simulink model "AMI_2_2_2"  (R2024b)
settings: Solver=FixedStepAuto  StartTime=0.0  StopTime=inf  FixedStep=0.01  RelTol=1e-3
libraries: simulink x10, instrumentseriallib x4
settings Model: Creator=wahaha  LastModifiedBy=chaiy
settings ModelReferenceCC: EnableRefExpFcnMdlSchedulingChecks=on
settings RTWCC: GPUComputeCapability=3.5

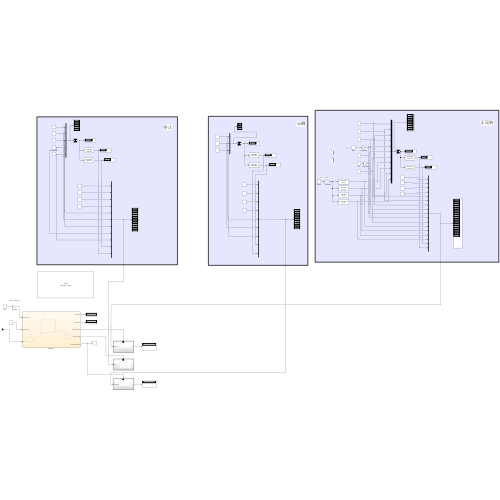
[thumbnail: Simulink's stored preview of the top-level diagram]
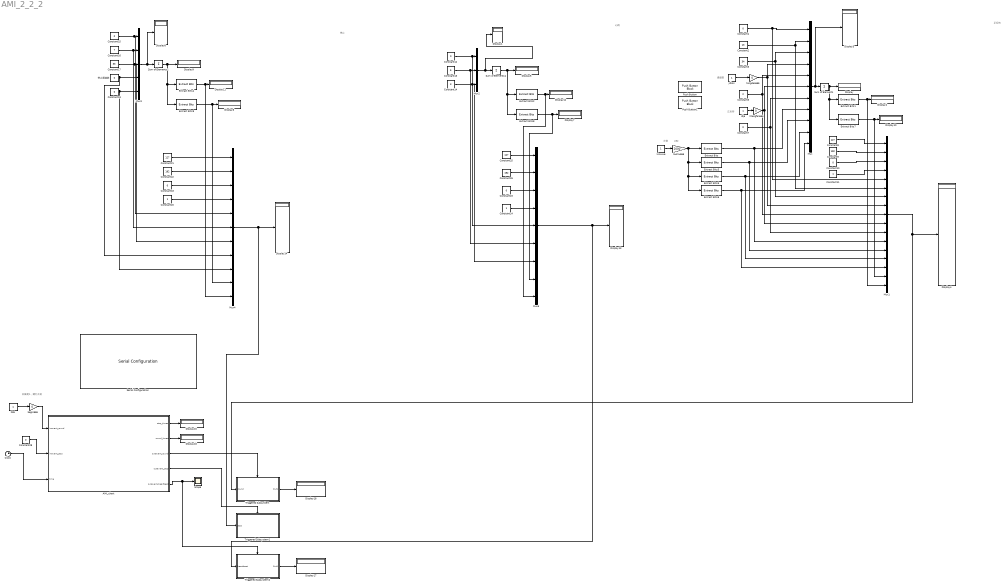
== system AMI_2_2_2 ==
  note: 通道数
  note: 正反转
  note: 步数
  note: 如果是1，螺钉开始
  note: U32
  note: 心跳
  note: 停止
  note: 正反转
  236 : Constant
  AMI_chart : Stateflow chart  TreatAsAtomicUnit=on
  Clock : Clock
  Constant{1,7,10,12,15,18..19,23} (8 alike) : Constant  Value=0  OutDataTypeStr=uint8
  Constant11 : Constant  OutDataTypeStr=uint8
  Constant13 : Constant  Value=5  OutDataTypeStr=uint8
  Constant14 : Constant  Value=3  OutDataTypeStr=uint8
  Constant16 : Constant  Value=7  OutDataTypeStr=uint8
  Constant17 : Constant  Value=33  OutDataTypeStr=uint8
  Constant2 : Constant  Value=13  OutDataTypeStr=uint8
  Constant20 : Constant  OutDataTypeStr=uint8
  Constant21 : Constant  Value=127  OutDataTypeStr=uint8
  Constant22 : Constant  Value=192  OutDataTypeStr=uint8
  Constant24 : Constant  OutDataTypeStr=uint8
  Constant25 : Constant  Value=127  OutDataTypeStr=uint8
  Constant26 : Constant  Value=192  OutDataTypeStr=uint8
  Constant28 : Constant  Value=0
  Constant3 : Constant  Value=34  OutDataTypeStr=uint8
  Constant5 : Constant  Value=2  OutDataTypeStr=uint8
  Constant8 : Constant  Value=127  OutDataTypeStr=uint8
  Constant9 : Constant  Value=192  OutDataTypeStr=uint8
  Display{,1..18} (19 alike) : Display
      Display settings: Format=hex (Stored Integer)
      Display1 settings: Format=hex (Stored Integer)
      Display10 settings: Format=hex (Stored Integer)
      Display11 settings: Format=hex (Stored Integer)
      Display12 settings: Format=hex (Stored Integer)
      Display13 settings: Format=hex (Stored Integer)
      Display14 settings: Format=hex (Stored Integer)
      Display15 settings: Format=decimal (Stored Integer)
      Display16 settings: Format=decimal (Stored Integer)
      Display17 settings: Format=decimal (Stored Integer)
      Display18 settings: Format=decimal (Stored Integer)
      Display2 settings: Format=hex (Stored Integer)
      Display3 settings: Format=hex (Stored Integer)
      Display4 settings: Format=hex (Stored Integer)
      Display5 settings: Format=hex (Stored Integer)
      Display6 settings: Format=hex (Stored Integer)
      Display7 settings: Format=hex (Stored Integer)
      Display8 settings: Format=hex (Stored Integer)
      Display9 settings: Format=hex (Stored Integer)
  Extract Bits : simulink/Logic and Bit Operations/Extract Bits  bitsToExtract=Range of bits  numBits=8  bitIdxRange=[24 31]  outScalingMode=Treat bit field as an integer
  Extract Bits1 : simulink/Logic and Bit Operations/Extract Bits  bitsToExtract=Lower half  numBits=8  bitIdxRange=[0 7]  outScalingMode=Treat bit field as an integer
  Extract Bits2 : simulink/Logic and Bit Operations/Extract Bits  bitsToExtract=Lower half  numBits=8  bitIdxRange=[0 7]  outScalingMode=Treat bit field as an integer
  Extract Bits3 : simulink/Logic and Bit Operations/Extract Bits  bitsToExtract=Range of bits  numBits=8  bitIdxRange=[16 23]  outScalingMode=Treat bit field as an integer
  Extract Bits4 : simulink/Logic and Bit Operations/Extract Bits  bitsToExtract=Lower half  numBits=8  bitIdxRange=[0 7]  outScalingMode=Treat bit field as an integer
  Extract Bits5 : simulink/Logic and Bit Operations/Extract Bits  bitsToExtract=Range of bits  numBits=8  bitIdxRange=[8 15]  outScalingMode=Treat bit field as an integer
  Extract Bits6 : simulink/Logic and Bit Operations/Extract Bits  bitsToExtract=Range of bits  numBits=8  bitIdxRange=[0 7]  outScalingMode=Treat bit field as an integer
  Extract Bits7 : simulink/Logic and Bit Operations/Extract Bits  bitsToExtract=Upper half  numBits=8  bitIdxRange=[0 7]  outScalingMode=Treat bit field as an integer
  Extract Bits8 : simulink/Logic and Bit Operations/Extract Bits  bitsToExtract=Upper half  numBits=8  bitIdxRange=[0 7]  outScalingMode=Treat bit field as an integer
  Extract Bits9 : simulink/Logic and Bit Operations/Extract Bits  bitsToExtract=Upper half  numBits=8  bitIdxRange=[0 7]  outScalingMode=Treat bit field as an integer
  Mux : Mux  Inputs=11
  Mux1 : Mux  Inputs=17
  Mux2 : Mux  Inputs=3
  Mux3 : Mux  Inputs=5
  Mux4 : Mux  Inputs=11
  Mux5 : Mux  Inputs=9
  Push Button : PushButtonBlock  ButtonText=round  OffValue=0.000000
  Push Button1 : PushButtonBlock  ButtonText=STOP  OffValue=0.000000
  Scope : Scope
  Serial Configuration : instrumentseriallib/Serial Configuration  Priority=-200000  PortSel=COM4  Port=COM4  ComPort=COM4  BaudRate=115200  DataBits=8  Parity=none  StopBits=1  ByteOrder=big-endian  FlowControl=none  Timeout=1  SimulateUsing=Interpreted execution  BlockInModel=on  aMode=1
  Sum of Elements : Sum  Inputs=+  CollapseDim=2  OutDataTypeStr=uint16  AccumDataTypeStr=uint16
  Sum of Elements1 : Sum  Inputs=+  CollapseDim=2  OutDataTypeStr=uint16  AccumDataTypeStr=uint16
  Sum of Elements2 : Sum  Inputs=+  CollapseDim=2  OutDataTypeStr=uint16  AccumDataTypeStr=uint16
  Triggered Subsystem : Subsystem  TreatAsAtomicUnit=on
  Triggered Subsystem1 : Subsystem  TreatAsAtomicUnit=on
  Triggered Subsystem2 : Subsystem  TreatAsAtomicUnit=on
  begin666 : Gain  Gain=0
  bushu666 : Gain  Gain=2000  ParamDataTypeStr=uint32  OutDataTypeStr=uint32
  idje : Constant  OutDataTypeStr=uint8
  jdkss : Constant  OutDataTypeStr=uint8
  kiswwe : Constant  OutDataTypeStr=uint32
  tongdao666 : Gain  Gain=0  ParamDataTypeStr=uint8  OutDataTypeStr=uint8
  zhengfan666 : Gain  Gain=0  ParamDataTypeStr=uint8  OutDataTypeStr=uint8
  停止通道数 : Constant  Value=0  OutDataTypeStr=uint8
  wires:
  Constant21/1 -> Mux4/1
  Constant5/1 -> Mux/5, Mux1/9
  Constant12/1 -> Mux5/5, Mux2/1
  Constant22/1 -> Mux4/2
  Constant19/1 -> Mux4/9, Mux3/5
  Constant24/1 -> Mux5/4
  Constant25/1 -> Mux5/1
  Constant10/1 -> Mux1/3
  Constant16/1 -> Mux4/6, Mux3/2
  Mux4/1 -> Triggered Subsystem1/1(stop), Display14/1
  Mux3/1 -> Sum of Elements2/1, Display8/1
  Mux5/1 -> Triggered Subsystem2/1(heartbeat), Display13/1
  Constant15/1 -> Mux4/5, Mux3/1
  Constant26/1 -> Mux5/2
  Constant23/1 -> Mux5/3
  停止通道数/1 -> Mux4/8, Mux3/4
  Constant20/1 -> Mux4/4
  Extract Bits7/1 -> Mux1/16, Display10/1
  Constant13/1 -> Mux5/6, Mux2/2
  idje/1 -> zhengfan666/1
  Constant17/1 -> Mux4/7, Mux3/3
  Sum of Elements/1 -> Extract Bits7/1, Extract Bits1/1, Display/1
  Constant14/1 -> Mux5/7, Mux2/3
  Constant3/1 -> Mux1/7, Mux/3
  Constant18/1 -> Mux4/3
  Constant1/1 -> Mux1/5, Mux/1
  Mux2/1 -> Display1/1, Sum of Elements1/1
  Constant9/1 -> Mux1/2
  Mux/1 -> Display3/1, Sum of Elements/1
  Constant11/1 -> Mux1/4
  Constant8/1 -> Mux1/1
  jdkss/1 -> tongdao666/1
  Constant2/1 -> Mux1/6, Mux/2
  Extract Bits1/1 -> Mux1/17, Display2/1
  Constant7/1 -> Mux/7, Mux1/11
  Mux1/1 -> Triggered Subsystem/1(round), Display4/1
  236/1 -> begin666/1
  Constant28/1 -> AMI_chart/2(inevent_stop)
  AMI_chart/1(stop_times) -> Display15/1
  AMI_chart/5(outevent_heartbeat) -> Triggered Subsystem2/Trigger, Scope/1
  Clock/1 -> AMI_chart/3(time)
  AMI_chart/2(round_times) -> Display16/1
  AMI_chart/3(outevent_round) -> Triggered Subsystem/Trigger
  AMI_chart/4(outevent_stop) -> Triggered Subsystem1/Trigger
  Triggered Subsystem2/1(Out1) -> Display17/1
  Triggered Subsystem/1(Out1) -> Display18/1
  kiswwe/1 -> bushu666/1
  Extract Bits/1 -> Mux1/12, Mux/8
  Extract Bits3/1 -> Mux1/13, Mux/9
  Extract Bits5/1 -> Mux1/14, Mux/10
  Extract Bits6/1 -> Mux1/15, Mux/11
  Extract Bits8/1 -> Mux5/8, Display7/1
  Extract Bits2/1 -> Mux5/9, Display12/1
  Sum of Elements1/1 -> Extract Bits8/1, Extract Bits2/1, Display5/1
  Extract Bits9/1 -> Mux4/10, Display6/1
  Extract Bits4/1 -> Mux4/11, Display11/1
  Sum of Elements2/1 -> Extract Bits9/1, Extract Bits4/1, Display9/1
  begin666/1 -> AMI_chart/1(inevent_round)
  tongdao666/1 -> Mux1/8, Mux/4
  zhengfan666/1 -> Mux/6, Mux1/10
  bushu666/1 -> Extract Bits6/1, Extract Bits5/1, Extract Bits3/1, Extract Bits/1

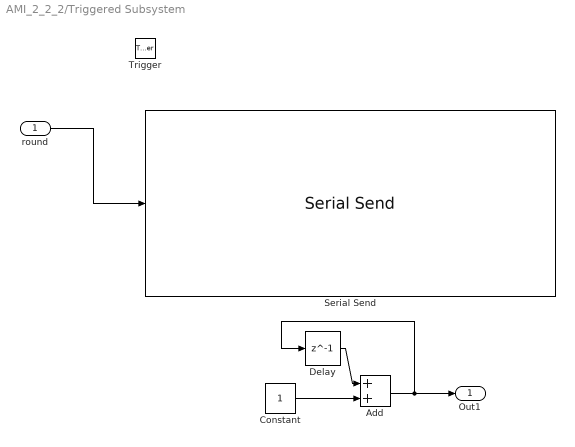
== system AMI_2_2_2/Triggered Subsystem ==
  round : Inport
  Trigger : TriggerPort  TriggerType=either  VariantControl=(inherit)
  Add : Sum
  Constant : Constant
  Delay : Delay  DelayLength=1  InitialCondition=0
  Serial Send : instrumentseriallib/Serial Send  Priority=1  PortSel=COM4  Port=COM4  ComPort=COM4  Header=[]  Terminator=<none>  CustomTerminator=[]  EnableBlockingMode=on  SimulateUsing=Interpreted execution  BlockInModel=on  aMode=1
  Out1 : Outport
  wires:
  round/1 -> Serial Send/1
  Delay/1 -> Add/1
  Constant/1 -> Add/2
  Add/1 -> Delay/1, Out1/1

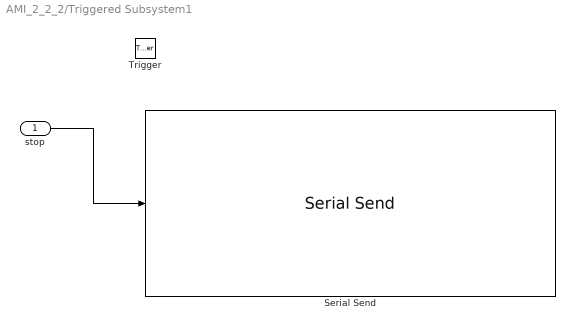
== system AMI_2_2_2/Triggered Subsystem1 ==
  stop : Inport
  Trigger : TriggerPort  TriggerType=either  VariantControl=(inherit)
  Serial Send : instrumentseriallib/Serial Send  Priority=1  PortSel=COM4  Port=COM4  ComPort=COM4  Header=[]  Terminator=<none>  CustomTerminator=[]  EnableBlockingMode=on  SimulateUsing=Interpreted execution  BlockInModel=on  aMode=1
  wires:
  stop/1 -> Serial Send/1

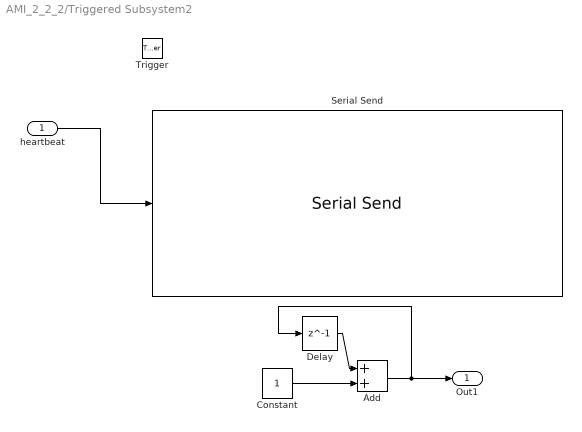
== system AMI_2_2_2/Triggered Subsystem2 ==
  heartbeat : Inport
  Trigger : TriggerPort  TriggerType=either  VariantControl=(inherit)
  Add : Sum
  Constant : Constant
  Delay : Delay  DelayLength=1  InitialCondition=0
  Serial Send : instrumentseriallib/Serial Send  Priority=1  PortSel=COM4  Port=COM4  ComPort=COM4  Header=[]  Terminator=<none>  CustomTerminator=[]  EnableBlockingMode=on  SimulateUsing=Interpreted execution  BlockInModel=on  aMode=1
  Out1 : Outport
  wires:
  heartbeat/1 -> Serial Send/1
  Add/1 -> Delay/1, Out1/1
  Constant/1 -> Add/2
  Delay/1 -> Add/1

== stateflow chart AMI_2_2_2/AMI_chart ==
  settings: executeAtInitialization=1
  state ini
    entry:
    start_time = time;
    during:
    if (~(rising(inevent_stop)))&&(~(rising(inevent_round)))&&(time - start_time >= 1)
    send(outevent_heartbeat);  % 定时触发
    start_time = time;   % 重置计时器
    end
  state round
    entry:
    round_times=round_times+1;
    send(outevent_round);
  state stop
    entry:
    stop_times=stop_times+1;
    send(outevent_stop);
  (default) -> ini
  ini -> round [order 1] : [rising(inevent_round)]
  ini -> stop [order 2] : [rising(inevent_stop)]
  round -> ini
  stop -> ini
  data: inevent_round input; inevent_stop input; stop_times output =0; round_times output =0; time input; start_time local =0
  events: outevent_round output EITHER_EDGE_EVENT; outevent_stop output EITHER_EDGE_EVENT; outevent_heartbeat output EITHER_EDGE_EVENT
